simulink model "conv_encoderdemo"  (Simulink 6.0)
settings: Solver=VariableStepDiscrete  StartTime=0.0  StopTime=500.0  RelTol=1e-3
PreLoadFcn:
  | %-- Initialize myTrellis structure
  | myTrellis.numInputSymbols = 8;
  | myTrellis.numOutputSymbols = 16;
  | myTrellis.numStates = 8;
  | 
  | myTrellis.nextStates = [0     1     2     3     0     1     2     3;
  |                         6     7     4     5     6     7     4     5;
  |                         1     0     3     2     1     0     3     2;
  |                         7     6     5     4     7     6     5     4;
  |                         2     3     0     1     2     3     0     1;
  |                         4     5     6     7     4     5     6     7;
  |                         3     2     1     0     3     2     1     0;
  |                         5     4     7     6     5     4     7     6];
  | myTrellis.outputs =  [0     2     4     6    10    12    14    16;
  |                       1     3     5     7    11    13    15    17;
  |                       0     2     4     6    10    12    14    16;
  |                       1     3     5     7    11    13    15    17;
  |                       0     2     4     6    10    12    14    16;
  |                       1     3     5     7    11    13    15    17;
  |                       0     2     4     6    10    12    14    16;
  |                       1     3     5     7    11    13    15    17];
libraries: dspsigops x3, commsink2 x2, commcnvcod2 x2, commrandsrc2 x1, simulink x1, dspindex x1
CloseFcn:
  | clear myTrellis convSigsOut;
settings Model: Creator=arodrigu  LastModifiedBy=mmclerno  BufferReuse=off  ProdHWDeviceType=Specified
settings DataIOCC: SaveOutput=off  SaveTime=off  SignalLoggingName=convSigsOut
settings OptimizationCC: BooleanDataType=off  OptimizeBlockIOStorage=off  BufferReuse=off  LocalBlockOutputs=off  MultiInstanced=off
settings FormatCC: IgnoreBidirectionalLines=off
settings HardwareCC: ProdHWDeviceType=Specified
settings CodeAppCC: MangleLength=5  SimulinkBlockComments=off
settings GRTTargetCC: TargetFcnLib=iso_c_tmw.mat

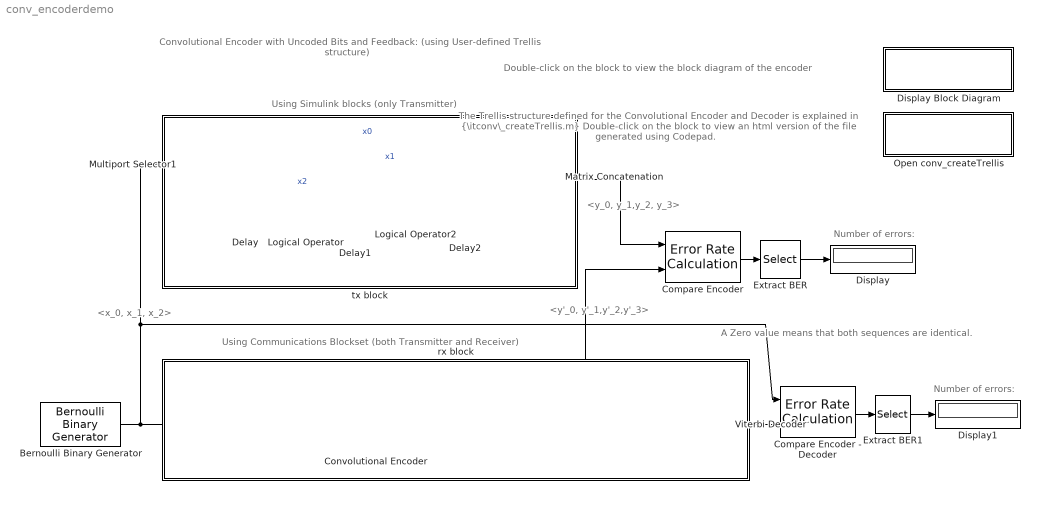
== system conv_encoderdemo ==
  note: <x_0, x_1, x_2>
  note: <y_0, y_1,y_2, y_3>
  note: Convolutional Encoder with Uncoded Bits and Feedback:
      | (using User-defined Trellis structure)
  note: <y'_0, y'_1,y'_2,y'_3>
  note: Using Simulink blocks (only Transmitter)
  note: Using Communications Blockset (both Transmitter and Receiver)
  note: The Trellis structure defined for the
      | Convolutional Encoder and Decoder
      | is explained in {\itconv\_createTrellis.m}
      | Double-click on the block to view an
      | html version of the file generated using
      | Codepad.
  note: Double-click on the block to view the
      | block diagram of the encoder
  note: A Zero value means that both
      | sequences are identical.
  note: Number of errors:
  note: Number of errors:
  Bernoulli Binary Generator : commrandsrc2/Bernoulli Binary Generator  P=0.5  seed=61  Ts=1/3  frameBased=on  sampPerFrame=3  orient=off
  Compare Encoder - Decoder : commsink2/Error Rate Calculation  N=34*3  st_delay=0  cp_mode=Entire frame  subframe=[]  PMode=Port  WsName=ErrorVec  RsMode2=off  stop=off  numErr=100  maxBits=1e6
  Compare Encoder : commsink2/Error Rate Calculation  N=0  st_delay=0  cp_mode=Entire frame  subframe=[]  PMode=Port  WsName=ErrorVec  RsMode2=off  stop=off  numErr=100  maxBits=1e6
  Convolutional Encoder : commcnvcod2/Convolutional Encoder  trellis=myTrellis % Stored in MATLAB Workspace  reset=None
  Delay : dspsigops/Delay  dly_unit=Samples  delay=1  ic_detail=off  dif_ic_for_ch=off  dif_ic_for_dly=off  ic=0  reset_popup=None
  Delay1 : dspsigops/Delay  dly_unit=Samples  delay=1  ic_detail=off  dif_ic_for_ch=off  dif_ic_for_dly=off  ic=0  reset_popup=None
  Delay2 : dspsigops/Delay  dly_unit=Samples  delay=1  ic_detail=off  dif_ic_for_ch=off  dif_ic_for_dly=off  ic=0  reset_popup=None
  Display : Display
  Display Block Diagram : Subsystem
      settings: OpenFcn=|
      | w=which([matlabroot filesep 'toolbox' filesep 'commblks' filesep 'commblksdemos' filesep 'conv_blckdiagram.jpg']);
      | 
      | if isempty(w)
      |     w = which('conv_blckdiagram.jpg');
      | end
      | if isempty(w)
      |     errordlg('Unable to find conv_blckdiagram.jpg file.');
      | end
      | X = imread(w);
      | [m,n] = size(X);
      | figure('Units','Pixels','Position',[200 200 n+2 m+2],'color','white');
      | imagesc(X); colormap gray;
      | set(gca,'Position',[0.01 0.01 1-0.02 1-0.02],'ytick',[0],'xtick',[0]);
      | set(gcf,'name','Block Diagram of Convolutional Encoder');
      | clear X m n w
      mask Display: disp('Display\nBlock Diagram')
  Display1 : Display
  Extract BER : Selector  InputPortWidth=3
  Extract BER1 : Selector  InputPortWidth=3
  Logical Operator : Logic  Operator=XOR  Inputs=3  AllPortsSameDT=off
  Logical Operator2 : Logic  Operator=XOR  AllPortsSameDT=off
  Matrix Concatenation : simulink/Math Operations/Matrix Concatenation  numInports=4  catMethod=Vertical
  Multiport Selector1 : dspindex/Multiport Selector  rowsOrCols=Rows  idxCellArray={1 2 3}  idxErrMode=Clip Index
  Open conv_createTrellis : Subsystem
      settings: OpenFcn=|
      | if exist([matlabroot filesep 'toolbox' filesep 'commblks' filesep 'commblksdemos' filesep 'html' filesep 'conv_createTrellis.html'])
      | 
      |     web([matlabroot filesep 'toolbox' filesep 'commblks' filesep 'commblksdemos' filesep 'html' filesep 'conv_createTrellis.html']);
      | 
      | else
      |     errordlg('Unable to find conv_createTrellis.html file.');
      | 
      | end
      mask Display: disp('Info')
  Viterbi Decoder : commcnvcod2/Viterbi Decoder  trellis=myTrellis % Stored in MATLAB Workspace  dectype=Hard Decision  nsdecb=4  tbdepth=34  opmode=Continuous  reset=off
  rx block : Subsystem
      mask Display: disp('')
  tx block : Subsystem
      mask Display: disp('')
  wires:
  Multiport Selector1/2 -> Logical Operator/1, Matrix Concatenation/2  "x1"
  Multiport Selector1/3 -> Logical Operator2/1, Matrix Concatenation/3  "x2"
  Delay/1 -> Logical Operator/2
  Logical Operator/1 -> Delay1/1
  Delay1/1 -> Logical Operator2/2
  Logical Operator2/1 -> Delay2/1
  Delay2/1 -> Logical Operator/3, Delay/1, Matrix Concatenation/4
  Convolutional Encoder/1 -> Viterbi Decoder/1, Compare Encoder/2
  Bernoulli Binary Generator/1 -> Convolutional Encoder/1, Compare Encoder - Decoder/1, Multiport Selector1/1
  Compare Encoder/1 -> Extract BER/1
  Matrix Concatenation/1 -> Compare Encoder/1
  Compare Encoder - Decoder/1 -> Extract BER1/1
  Viterbi Decoder/1 -> Compare Encoder - Decoder/2
  Multiport Selector1/1 -> Matrix Concatenation/1  "x0"
  Extract BER/1 -> Display/1
  Extract BER1/1 -> Display1/1

== system conv_encoderdemo/Display Block Diagram ==
  note: This sub-system is empty.

== system conv_encoderdemo/Open conv_createTrellis ==
  note: This sub-system is empty.

== system conv_encoderdemo/rx block ==

== system conv_encoderdemo/tx block ==
